simulink model "ZETAConverter"  (R2017a)
settings: Solver=ode23tb  StartTime=0.0  StopTime=1  FixedStep=1e-5  MaxStep=1e-4  RelTol=1e-3
libraries: powerlib x17
settings Model: Creator=acer  LastModifiedBy=acer

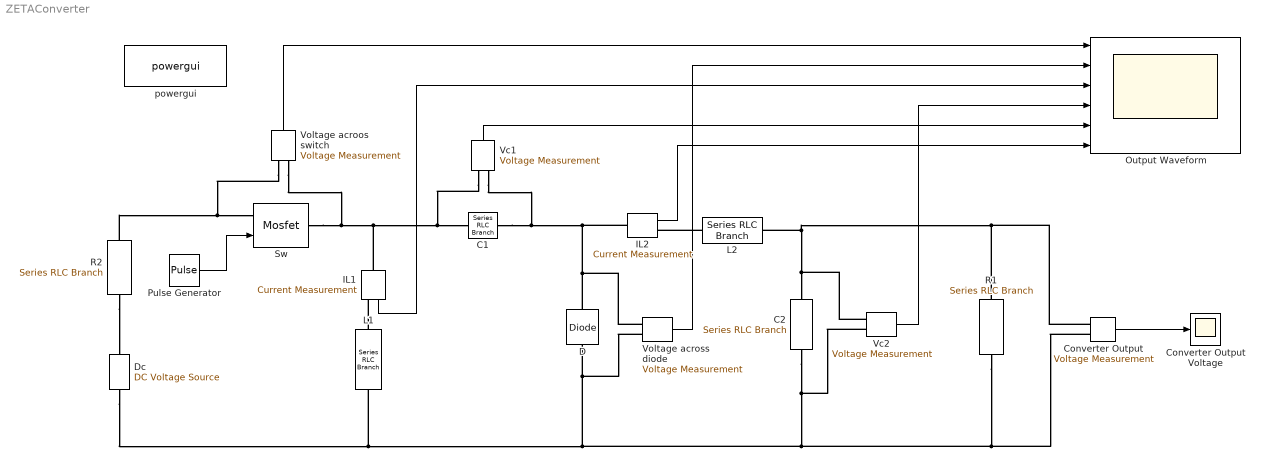
== system ZETAConverter ==
  C1 : powerlib/Elements/Series RLC Branch  LConnTagsString=__new0  RConnTagsString=__new0  BranchType=C  Resistance=100  Inductance=1e-3  SetiL0=off  InitialCurrent=0  Capacitance=114e-6  Setx0=off  InitialVoltage=0  Measurements=None
  C2 : powerlib/Elements/Series RLC Branch  LConnTagsString=__new0  RConnTagsString=__new0  BranchType=C  Resistance=1  Inductance=1e-3  SetiL0=off  InitialCurrent=0  Capacitance=12e-6  Setx0=off  InitialVoltage=0  Measurements=None
  Converter Output : powerlib/Measurements/Voltage Measurement  PhasorSimulation=off  OutputType=Complex  PSBequivalent=0
  Converter Output Voltage : Scope
  D : powerlib/Power Electronics/Diode  Ron=0.001  Lon=0  Vf=.05  IC=0  UseSnubber=off  Rs=500  Cs=250e-9  Measurements=off
  Dc : powerlib/Electrical Sources/DC Voltage Source  Amplitude=15  Measurements=Voltage
  IL1 : powerlib/Measurements/Current Measurement  PhasorSimulation=off  OutputType=Complex  PSBequivalent=0
  IL2 : powerlib/Measurements/Current Measurement  PhasorSimulation=off  OutputType=Complex  PSBequivalent=0
  L1 : powerlib/Elements/Series RLC Branch  LConnTagsString=__new0  RConnTagsString=__new0  BranchType=L  Resistance=1  Inductance=.28571e-3  SetiL0=off  InitialCurrent=0  Capacitance=1e-6  Setx0=off  InitialVoltage=0  Measurements=None
  L2 : powerlib/Elements/Series RLC Branch  LConnTagsString=__new0  RConnTagsString=__new0  BranchType=L  Resistance=1  Inductance=.28571e-3  SetiL0=off  InitialCurrent=0  Capacitance=1e-6  Setx0=off  InitialVoltage=0  Measurements=None
  Output Waveform : Scope  NumInputPorts=6
  Pulse Generator : DiscretePulseGenerator  PulseType=Time based  Period=2e-5  PulseWidth=57.5
  R1 : powerlib/Elements/Series RLC Branch  LConnTagsString=__new0  RConnTagsString=__new0  BranchType=R  Resistance=20  Inductance=1e-3  SetiL0=off  InitialCurrent=0  Capacitance=1e-6  Setx0=off  InitialVoltage=0  Measurements=None
  R2 : powerlib/Elements/Series RLC Branch  LConnTagsString=__new0  RConnTagsString=__new0  BranchType=R  Resistance=1e-12  Inductance=1e-3  SetiL0=off  InitialCurrent=0  Capacitance=1e-6  Setx0=off  InitialVoltage=0  Measurements=None
  Sw : powerlib/Power Electronics/Mosfet  Ron=0.1  Lon=0  Rd=0.01  Vfd=0  IC=0  Rs=1e5  Cs=inf  Measurements=off
  Vc1 : powerlib/Measurements/Voltage Measurement  PhasorSimulation=off  OutputType=Complex  PSBequivalent=0
  Vc2 : powerlib/Measurements/Voltage Measurement  PhasorSimulation=off  OutputType=Complex  PSBequivalent=0
  Voltage acroos switch : powerlib/Measurements/Voltage Measurement  PhasorSimulation=off  OutputType=Complex  PSBequivalent=0
  Voltage across diode : powerlib/Measurements/Voltage Measurement  PhasorSimulation=off  OutputType=Complex  PSBequivalent=0
  powergui : powerlib/powergui  Priority=1  SimulationMode=Continuous  SampleTime=5e-5  frequency=50  Iterations=50  frequencyindice=0  Pbase=100e6  ErrMax=1e-4  UnitsV=kV  UnitsW=MW  buscounter=0  FunctionMessages=off  echomessages=off  EnableUseOfTLC=off  CurrentSourceSwitches=off  DisableSnubberDevices=off  DisableRonSwitches=off  DisableVfSwitches=off  DisplayEquations=off  SolverType=Tustin/Backward Euler (TBE)  Interpol=off  ExternalGateDelay=off  methode=off  Ts=100  x0status=blocks  SPID=on  SwTol=0  HookPort=off  RestoreLinks=warning  ResistiveCurrentMeasurement=off  Frange=[0:2:500]  Ylog=off  Xlog=on  ShowGrid=off  save=off  variable=ZData  structure=0  ZoomFFT=on  StartTime=0.0  cycles=1  DisplayStyle=1  fundamental=60  FreqAxis=off  MaxFrequency=1000  frequencyindicesteady=1  RmsSteady=1  display=off
  wires:
  Pulse Generator/1 -> Sw/1
  Converter Output/1 -> Converter Output Voltage/1
  Voltage acroos switch/1 -> Output Waveform/1
  Voltage across diode/1 -> Output Waveform/2
  Vc2/1 -> Output Waveform/4
  IL1/1 -> Output Waveform/3
  IL2/1 -> Output Waveform/6
  Vc1/1 -> Output Waveform/5
  connections:
  Sw/RConn1 -- Voltage acroos switch/LConn2 -- Vc1/LConn1 -- C1/LConn1 -- IL1/LConn1
  Vc2/LConn2 -- C2/RConn1 -- Converter Output/LConn2 -- R1/RConn1 -- Dc/LConn1 -- L1/RConn1 -- Voltage across diode/LConn2 -- D/LConn1
  L2/RConn1 -- Vc2/LConn1 -- C2/LConn1 -- Converter Output/LConn1 -- R1/LConn1
  C1/RConn1 -- Vc1/LConn2 -- Voltage across diode/LConn1 -- D/RConn1 -- IL2/LConn1
  R2/RConn1 -- Dc/RConn1
  R2/LConn1 -- Voltage acroos switch/LConn1 -- Sw/LConn1
  L1/LConn1 -- IL1/RConn1
  L2/LConn1 -- IL2/RConn1
